simulink library "pdc_grc"  (R2024a)
settings: Solver=VariableStepAuto  StartTime=0.0  StopTime=10.0  RelTol=1e-3
undefined symbols (not defined in the file or in its folder): ENUM_IVTROPMODE_ASCHI, ENUM_IVTROPMODE_ASCLO, ENUM_IVTROPMODE_DTCYCTRL, ENUM_IVTROPMODE_FW, ENUM_IVTROPMODE_IVTROFF, KASC_DecDuty_value, KASC_OpenTime_s, KCCM_ASCSwitchEna_flg, KDSM_bIvtrTarHiDebug_flg, KDSM_DiagSpdH_rpm, KDSM_DiagSpdL_rpm, KeMCCR_b_UseMeasCrntDTC, KeSVMR_b_UseStrictClamp, KeSVMR_FullDTCCurr_A, KeSVMR_PWMPrd_cnt, KeSVMR_StrClampMaxDuty_pct, KeSVMR_StrClampMinDuty_pct, KeSVMR_t_DeadTime, KeSVMR_t_MinPulseWidth, KOSP_IvtrTarMor_enum_ovrdflg, KOSP_IvtrTarMor_enum_ovrdval, KPDC_facScalePWM_C, KPDC_FWCnt_C, KPDC_nPosnErrMaxSpd_C, StIvtrMod, StMotMod
libraries: simulink x18, GRC_Lib x6
(part 3 of 3)

== stateflow chart pdc_grc/PDC/PWMCalculation/Inverter Control /SS_SafetyShutdown_Ctrl ==
  state Normal
    %MCU is in normal state.
    en:
    SS_u8_SafetySts_null = ENUM_IVTROPMODE_DTCYCTRL;
    note: % Spd大于某值，才能由normal转移到上桥臂或下桥臂短路
  note: % f32_EntASC_rpm--->进入主动短路
      |     f32_ExtASC_rpm--->退出主动短路
      |     低速关管(freewheel)，高速主动短路(ASC)
  note: %严重故障且Spd<=某一转速
      | (此时反电动势较小)
  state ASC_Up
    %The up bridge is short circuit
    en:
    SS_u8_SafetySts_null = ENUM_IVTROPMODE_ASCHI;
  state FWL
    %The IGBT bridge is off
    en:
    SS_u8_SafetySts_null = ENUM_IVTROPMODE_FW;
    note: 进入Freewheel都是Spd<=某一转速
  note: % ASC时候一般默认下桥臂主动短路
  state ASC_Dwn
    %The down bridge is short circuit
    en:
    SS_u8_SafetySts_null = ENUM_IVTROPMODE_ASCLO;
  (default) -> Normal
  Normal -> ASC_Up [order 2] : [(FaultLevel2==1)...
      | &&(SPI1_f32_MeclSpd_rpm>=f32_EntASC_rpm)...
      | &&(SPI2_b1_IGBTDwnErr_null>=1)...
      | &&(SPI2_b1_IGBTUpErr_null<=0)...
      | &&(Diag1_bOverCurrent == 0)]
  FWL -> Normal [order 3] : [DIAG_B1_CPLDFLTCLC_NULL>=1]
  Normal -> FWL [order 3] : [FaultLevel2==1]
  Normal -> ASC_Dwn [order 1] : [(FaultLevel2==1)...
      | &&(SPI1_f32_MeclSpd_rpm>=f32_EntASC_rpm)...
      | &&(SPI2_b1_IGBTDwnErr_null<=0)...
      | &&(Diag1_bOverCurrent == 0)]
  FWL -> ASC_Up [order 2] : [(SPI1_f32_MeclSpd_rpm>=f32_EntASC_rpm)...
      | &&(SPI2_b1_IGBTUpErr_null<=0)...
      | &&(SPI2_b1_IGBTDwnErr_null>=1)...
      | &&(Diag1_bOverCurrent == 0)]
  ASC_Up -> FWL [order 1] : [(SPI1_f32_MeclSpd_rpm<=f32_ExtASC_rpm)]
  FWL -> ASC_Dwn [order 1] : [(SPI1_f32_MeclSpd_rpm>=f32_EntASC_rpm)...
      | &&(SPI2_b1_IGBTDwnErr_null<=0)...
      | &&(Diag1_bOverCurrent == 0)]
  ASC_Dwn -> FWL [order 1] : [(SPI1_f32_MeclSpd_rpm<=f32_ExtASC_rpm)]
  ASC_Dwn -> ASC_Up [order 2] : [(SPI2_b1_IGBTUpErr_null<=0)...
      | &&(SPI2_b1_IGBTDwnErr_null>=1)...
      | &&(Diag1_bOverCurrent == 0)]
  ASC_Up -> ASC_Dwn [order 2] : [(SPI2_b1_IGBTUpErr_null>=1)...
      | &&(SPI2_b1_IGBTDwnErr_null<=0)...
      | &&(Diag1_bOverCurrent == 0)]
  data: SPI1_f32_MeclSpd_rpm input single; SPI2_b1_IGBTUpErr_null input boolean; SPI2_b1_IGBTDwnErr_null input boolean; SS_u8_SafetySts_null output uint8; FaultLevel2 input boolean; Diag1_bOverCurrent input; DIAG_B1_CPLDFLTCLC_NULL input boolean; f32_EntASC_rpm input single; f32_ExtASC_rpm input single; ENUM_IVTROPMODE_ASCHI parameter; ENUM_IVTROPMODE_ASCLO parameter; ENUM_IVTROPMODE_DTCYCTRL parameter; ENUM_IVTROPMODE_FW parameter

== stateflow chart pdc_grc/PDC/PWMCalculation/Inverter Control /SS_SafetyShutdown_Ctrl1 ==
  state Normal
    %MCU is in normal state.
    en:
    SS_u8_SafetySts_null=StIvtrMod.StIvtrModDtcyCtrl;
    note: % Spd大于某值，才能由normal转移到上桥臂或下桥臂短路
  note: % f32_EntASC_rpm--->进入主动短路
      |     f32_ExtASC_rpm--->退出主动短路
      |     低速关管(freewheel)，高速主动短路(ASC)
  note: %严重故障且Spd<=某一转速
      | (此时反电动势较小)
  state FWL
    %The IGBT bridge is off
    en:
    SS_u8_SafetySts_null=StIvtrMod.StIvtrModFW;
    note: 进入Freewheel都是Spd<=某一转速
  note: % ASC时候一般默认下桥臂主动短路
  state ASC
    state Open
      (default) -> (junction 73) : {
          | OpTimer = 0;
          | }
      Open -> (junction 73) [order 1] : {OpTimer= OpTimer + single(0.0001);}
      (junction 73) -> (junction 74) : {
          | VOSP_PWMEna_flg = 0;
          | }
    state ASC
      (default) -> (junction 82)
      ASC.ASC -> (junction 82)
      (junction 82) -> (junction 83) [order 1] : [VHSPI_IGBTDwnFlt_flg == 0]
      (junction 82) -> (junction 84) [order 2] : {
          | ActDutyU = 1;
          | ActDutyV = 1;
          | ActDutyW = 1;
          | }
      (junction 83) -> (junction 85) : {
          | ActDutyU = 0;
          | ActDutyV = 0;
          | ActDutyW = 0;
          | }
      (junction 85) -> (junction 84)
      (junction 84) -> (junction 86) : {VOSP_ASCEna_flg = 1;}
    state Switch
      (default) -> (junction 60) : {
          | VOSP_PWMEna_flg = 1;
          | ActDutyU = 0.5;
          | ActDutyV = 0.5;
          | ActDutyW = 0.5;
          | }
      Switch -> (junction 60) [order 1] : {
          | ActDutyU = ActDutyU-Duty;
          | ActDutyV = ActDutyV-Duty;
          | ActDutyW = ActDutyW-Duty;
          | }
      (junction 60) -> (junction 61) [order 1] : [ActDutyU > 0]
      (junction 61) -> (junction 63) : {
          | ASCEna = 0;
          | }
      (junction 60) -> (junction 62) [order 2] : {
          | ActDutyU = 0;
          | ActDutyV = 0;
          | ActDutyW = 0;
          | ASCEna =1;
          | }
      (junction 63) -> (junction 62)
      (junction 62) -> (junction 64)
    Open -> ASC.ASC [order 2] : [KCCM_ASCSwitchEna_flg ==0]
    Open -> Switch [order 1] : [OpTimer > OpenTime_s]
    Switch -> ASC.ASC [order 1] : [ASCEna == 1]
  (default) -> Normal
  Normal -> ASC [order 2] : [(FaultLevel2==1)...
      | &&(SPI1_f32_MeclSpd_rpm>=f32_EntASC_rpm)...
      | &&(SPI2_b1_IGBTDwnErr_null<=0)...
      | &&(Diag1_bOverCurrent == 0)]
  FWL -> Normal : [DIAG_B1_CPLDFLTCLC_NULL>=1]
  Normal -> FWL [order 1] : [(FaultLevel2==1)...
      | &&(SPI1_f32_MeclSpd_rpm<=f32_ExtASC_rpm)]
  ASC -> FWL : [(SPI1_f32_MeclSpd_rpm<=f32_ExtASC_rpm)]
  data: SPI1_f32_MeclSpd_rpm input single; SPI2_b1_IGBTUpErr_null input boolean; SPI2_b1_IGBTDwnErr_null input boolean; SS_u8_SafetySts_null output Enum: StIvtrMod; FaultLevel2 input boolean; Diag1_bOverCurrent input; DIAG_B1_CPLDFLTCLC_NULL input boolean; f32_EntASC_rpm input single; f32_ExtASC_rpm input single

== stateflow chart pdc_grc/PDC/PWMCalculation/PWMCmdCtrlEnable/ThreePhaseSC1/ASC ==
  state Open
    (default) -> (junction 5) : {
        | OpTimer = 0;
        | }
    Open -> (junction 5) [order 1] : {OpTimer= OpTimer + single(0.0001);}
    (junction 5) -> (junction 14) : {
        | PDC_Ivtr1ModCmd = 0;
        | ActDutyU = 0.5;
        | ActDutyV = 0.5;
        | ActDutyW = 0.5;
        | }
  state ASC
    (default) -> (junction 33)
    (junction 33) -> (junction 49) [order 1] : [PWMType == 2]
    ASC -> (junction 33)
    (junction 33) -> (junction 39) [order 2] : {
        | PDC_Ivtr1ModCmd=3;
        | ActDutyU = 1;
        | ActDutyV = 1;
        | ActDutyW = 1;
        | }
    (junction 49) -> (junction 51) : {
        | PDC_Ivtr1ModCmd=2;
        | ActDutyU = 0;
        | ActDutyV = 0;
        | ActDutyW = 0;
        | }
    (junction 51) -> (junction 39)
    (junction 39) -> (junction 54)
  state Switch
    (default) -> (junction 18) : {
        | PDC_Ivtr1ModCmd = 1;
        | ActDutyU = 0.5;
        | ActDutyV = 0.5;
        | ActDutyW = 0.5;
        | }
    Switch -> (junction 18) [order 1] : {
        | ActDutyU = ActDutyU-Duty;
        | ActDutyV = ActDutyV-Duty;
        | ActDutyW = ActDutyW-Duty;
        | }
    (junction 18) -> (junction 21) [order 1] : [ActDutyU > 0]
    (junction 21) -> (junction 23) : {
        | ASCEna = 0;
        | }
    (junction 18) -> (junction 26) [order 2] : {
        | ActDutyU = 0;
        | ActDutyV = 0;
        | ActDutyW = 0;
        | ASCEna =1;
        | }
    (junction 23) -> (junction 26)
    (junction 26) -> (junction 29)
  (default) -> Open
  Open -> ASC [order 2] : [KCCM_ASCSwitchEna_flg ==0]
  Open -> Switch [order 1] : [OpTimer > OpenTime_s]
  Switch -> ASC [order 1] : [ASCEna == 1]
  data: KCCM_ASCSwitchEna_flg input; ActDutyU output; ActDutyV output; ActDutyW output; Duty input; OpTimer local single =0; OpenTime_s input; PWMType input; PDC_Ivtr1ModCmd output uint8; ASCEna local boolean

== stateflow chart pdc_grc/PDC/PWMCalculation/PWMCmdCtrlEnable/ThreePhaseSC/ASC2 ==
  (default) -> (junction 150)
  (junction 150) -> (junction 153) [order 1] : [ASCPWMEna == 0]
  (junction 150) -> (junction 124) [order 2]
  (junction 153) -> (junction 155) : {
      | ActDuty = Duty;
      | PDC_Ivtr1ModCmd = 1;
      | }
  (junction 124) -> (junction 127) [order 1] : [Counter<fwCnt]
  (junction 124) -> (junction 132) [order 2]
  (junction 127) -> (junction 126) : {
      | Counter++;
      | PDC_Ivtr1ModCmd = 0;
      | ActDuty[0] = 0.5;
      | ActDuty[1] = 0.5;
      | ActDuty[2] = 0.5;
      | }
  (junction 132) -> (junction 135) [order 1] : [PWMType == 2]
  (junction 132) -> (junction 128) [order 2] : {
      | PDC_Ivtr1ModCmd=3;
      | ActDuty[0] = 1;
      | ActDuty[1] = 1;
      | ActDuty[2] = 1;
      | }
  (junction 135) -> (junction 133) : {
      | PDC_Ivtr1ModCmd=2;
      | ActDuty[0] = 0;
      | ActDuty[1] = 0;
      | ActDuty[2] = 0;
      | }
  (junction 133) -> (junction 128)
  (junction 126) -> (junction 133)
  (junction 155) -> (junction 126)
  (junction 128) -> (junction 138)
  data: PWMType input; ASCPWMEna input; PDC_Ivtr1ModCmd output uint8; Counter local uint8 =0; fwCnt input uint8; ActDuty output single size=[1 3]; Duty input

== stateflow chart pdc_grc/PDC/WorkTimeCalculation/Overmodulation/Overmodulation ==
  (default) -> (junction 20) : {
      | T_total = TM_Vector_Component_T1_p + TM_Vector_Component_T2_p;
      | }
  (junction 20) -> (junction 21) [order 1] : [T_total > Duty_Max]
  (junction 21) -> (junction 22) [order 1] : [ (TM_Vector_Component_T1_p <=Duty_Max) && (TM_Vector_Component_T2_p <= Duty_Max) ]
  (junction 20) -> (junction 19) [order 2] : {
      |  TM_Vector_Component_T1 = TM_Vector_Component_T1_p;
      |  TM_Vector_Component_T2 = TM_Vector_Component_T2_p;
      | }
  (junction 21) -> (junction 18) [order 2]
  (junction 22) -> (junction 28) : {
      |   T_temp = Duty_Max / T_total ;
      |   TM_Vector_Component_T1 = TM_Vector_Component_T1_p * T_temp ;
      |   TM_Vector_Component_T2 = TM_Vector_Component_T2_p * T_temp ;
      |  }
  (junction 18) -> (junction 23) [order 1] : [ (TM_Vector_Component_T1_p >Duty_Max) && (TM_Vector_Component_T1_p > TM_Vector_Component_T2_p) ]
  (junction 18) -> (junction 24) [order 2]
  (junction 23) -> (junction 27) : {
      |  TM_Vector_Component_T1 = Duty_Max;
      |  TM_Vector_Component_T2 = 0;
      | }
  (junction 24) -> (junction 25) [order 1] : [ (TM_Vector_Component_T2_p >Duty_Max ) && (TM_Vector_Component_T2_p > TM_Vector_Component_T1_p) ]
  (junction 24) -> (junction 30) [order 2] : {
      |   TM_Vector_Component_T1 = Duty_Max/2;
      |   TM_Vector_Component_T2 = Duty_Max/2;
      | }
  (junction 25) -> (junction 26) : {
      |  TM_Vector_Component_T1 = 0;
      |  TM_Vector_Component_T2 = Duty_Max;
      | }
  (junction 30) -> (junction 19)
  (junction 26) -> (junction 30)
  (junction 27) -> (junction 26)
  (junction 28) -> (junction 27)
  (junction 19) -> (junction 29)
  data: TM_Vector_Component_T1 output; TM_Vector_Component_T2 output; T_total local single; Duty_Max input; TM_Vector_Component_T1_p input; TM_Vector_Component_T2_p input; T_temp local single
